simulink model "MUDV_projekt"  (R2023a)
settings: Solver=ode23tb  StartTime=0.0  StopTime=20  FixedStep=.001  RelTol=2e-1  EnableMultiTasking=on
InitFcn:
  | v=version('-release');
  | if (str2num(v(1:end-1)) > 2021)
  | set_param('MUDV_projekt/Passenger Vehicle/Body, suspension and tires/MacPherson Front Suspension Solid Axle Rear Suspension/independent Suspensions - MacPherson','NumWhlsByAxl','2');
  | set_param('MUDV_projekt/Passenger Vehicle/Body, suspension and tires/MacPherson Front Suspension Solid Axle Rear Suspension/Solid Axle Suspension - Coil Spring','NumWhlsByAxl','2');
  | end
StartFcn:
  | %tic
StopFcn:
  | %toc
model workspace (MAT data in the model file):
  AxlIxx = 62.3745166667
  AxlM = 160
  Cps = 2
  Cz = 5565.2246438
  CzWhlAxl = 11490.971257
  DCT_Param : object (value not decoded)
  DLCXref = [0 7.35 7.45 18 33 33.5 45 50 60]
  DLCYref = [0 0 -4.5 -4.35 -3.75 1.25 1 0 0]
  EngRevLim = 7000
  F0z = [2886 2907]
  F0zWhlAxl = 2907
  Hmax = 0.25
  Kz = 52451.0065793
  KzWhlAxl = 138031.612078
  NCyl = 6
  Pedal_Positions = [0.1 0.4 0.5 0.9]
  Pstd = 101325
  Rair = 287
  SUS : object (value not decoded)
  Sig : Simulink.Signal (value not decoded)
  Sig1 : Simulink.Signal (value not decoded)
  Trans : object (value not decoded)
  Tstd = 293.15
  VEH : object (value not decoded)
  Vd = 0.00346
  WH : Mass (value not decoded)
  dt3D = 0.05
  f_air = [0 0 0 0 0 0 0 0 0 0 0 0 ... (256 elements, 16x16)]
  f_co = [0 0 0 0 0 0 0 0 0 0 0 0 ... (256 elements, 16x16)]
  f_co2 = [0 0 0 0 0 0 0 0 0 0 0 0 ... (256 elements, 16x16)]
  f_eff = [352.135682859 352.135682859 320.724378192 303.655312657 295.930136708 291.240087194 291.240271258 291.240312459 291.240275452 291.240198499 291.240100781 291.240018769 ... (256 elements, 16x16)]
  f_fuel = [0 0 0 0 0 0 0 0 0 0 0 0 ... (256 elements, 16x16)]
  f_hc = [0 0 0 0 0 0 0 0 0 0 0 0 ... (256 elements, 16x16)]
  f_nox = [0 0 0 0 0 0 0 0 0 0 0 0 ... (256 elements, 16x16)]
  f_pm = [0 0 0 0 0 0 0 0 0 0 0 0 ... (256 elements, 16x16)]
  f_susp_axl_bp = [1 2]
  f_susp_dz_bp = [-0.325022776267 -0.315022776267 -0.305022776267 -0.205022776267 -0.105022776267 -0.00502277626717 0.0949772237328 0.194977223733 0.204977223733 0.214977223733]
  f_susp_dzdot_bp = [-3 -0.3 -0.2 -0.1 0 0.1 0.2 0.3 3]
  f_susp_fmz = [-144070.391448 -93629.24037 -75929.1118915 -20630.5828179 -15385.48216 -10140.3815021 -4895.28084414 349.819813785 -31916.3973792 18437.6709544 -83996.1993354 -33555.0482577 ... (43920 elements, 10x9x61x2x4)]
  f_susp_geom = [0 0 0 0 0 0 0 0 0 0 0 0 ... (3660 elements, 10x61x2x3)]
  f_susp_strgdelta_bp = [-0.523598775598 -0.506145483078 -0.488692190558 -0.471238898038 -0.453785605519 -0.436332312999 -0.418879020479 -0.401425727959 -0.383972435439 -0.366519142919 -0.349065850399 -0.331612557879 ... (61 elements, 1x61)]
  f_tbrake = [0 76.8593923996 105.140482948 131.533638111 157.926793274 176.658631717 176.65727296 176.656856686 176.656879077 176.657093756 176.657404516 176.65772406 ... (256 elements, 16x16)]
  f_tbrake_n_bpt = [0 649.519052838 912.419621844 1175.32019085 1438.22075986 1701.12132886 1964.02189787 2226.92246687 2489.82303588 2752.72360489 3015.62417389 3278.5247429 ... (16 elements, 1x16)]
  f_tbrake_t_bpt = [0 34.6410161514 61.0341713143 87.4273264773 113.82048164 140.213636803 166.606791966 192.999947129 219.393102292 245.786257455 272.179412618 298.572567781 ... (16 elements, 1x16)]
  f_texh = [766.752464599 766.752464599 786.17542386 801.679939032 884.591982581 910.574397722 910.571871054 910.570774534 910.570601632 910.570821151 910.571247242 910.571639815 ... (256 elements, 16x16)]
  f_twc_eff_co = [0.17 0.25 0.45 0.99 0.99 0.99 0.99]
  f_twc_eff_hc = [0.21 0.375 0.75 0.98 0.98 0.98 0.98]
  f_twc_eff_lam = [0.909090909 0.944055944 0.979020979 1 1.013986014 1.048951049 1.083916084]
  f_twc_eff_nox = [0.98 0.98 0.98 0.97 0.05 0.02 0]
  numWheel = 4
symbols that are objects in the model workspace (value not decoded): VEH
libraries: sharedtransform x3, autolibutils x3, sim3dlib x2, vehdynlibsuspension x2, shared6dof x2, vehdynlibeom x1, vehdynlibtirecommon x1, vehdynlibtire x1, vehdynlibsteering x1, vehdynlibsens x1, sim3dautolib x1
(part 2 of 4)

== system MUDV_projekt/ Reference Generator  ==
  VehFdbk : Inport
  Add : Sum
  Bus Creator1 : BusCreator  Inputs=3
  Bus Selector : BusSelector  OutputSignals=Body.InertFrm.Cg.Disp.X
  DLC Reference : MATLAB Function  TreatAsAtomicUnit=on
  Manual Switch : ManualSwitch  CurrentSetting=0
  Rate Limiter : RateLimiter  RisingSlewLimit=10  FallingSlewLimit=-10  SampleTimeMode=inherited
  Scope : Scope
  Unit Delay : UnitDelay  SampleTime=1e-3  HasFrameUpgradeWarning=on
  X_offset : Constant  Value=30
  Y_offset : Constant  Value=0.2
  "km/h -> m/s" : Gain  Gain=1/3.6
  vxRef : Step  Time=0.1  After=50  SampleTime=0
  vxRef1 : Step  Time=0.1  After=20  SampleTime=10
  VehRef : Outport
  wires:
  Bus Creator1/1 -> VehRef/1
  DLC Reference/2(YRef) -> Bus Creator1/3  "LtrlRef"
  DLC Reference/1(YawRef) -> Bus Creator1/2  "YawRef"
  VehFdbk/1 -> Bus Selector/1
  Bus Selector/1 -> Unit Delay/1  "<X>"
  Y_offset/1 -> DLC Reference/3(Y_offset)
  "km/h -> m/s"/1 -> Scope/1, Bus Creator1/1  "LngRef"
  Unit Delay/1 -> DLC Reference/1(X)
  Rate Limiter/1 -> "km/h -> m/s"/1
  X_offset/1 -> DLC Reference/2(X_offset)
  Manual Switch/1 -> Rate Limiter/1
  vxRef/1 -> Manual Switch/2, Add/2
  Add/1 -> Manual Switch/1
  vxRef1/1 -> Add/1

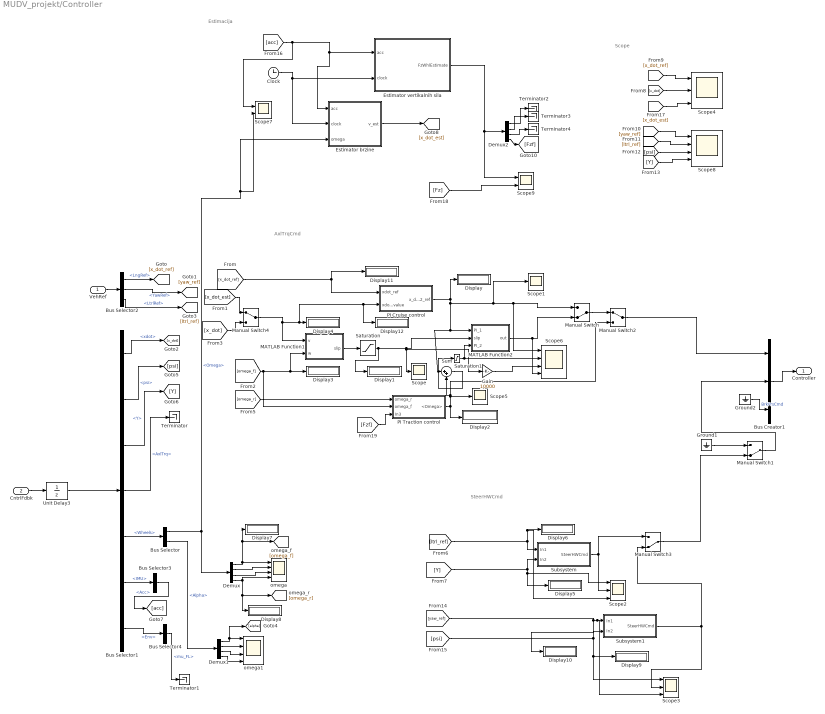
== system MUDV_projekt/Controller ==
  note: Estimacija
  note: Scope
  note: AxlTrqCmd
  note: SteerHWCmd
  VehRef : Inport
  CntrlFdbk : Inport  Port=2
  Bus Creator1 : BusCreator  Inputs=3
  Bus Selector : BusSelector  OutputSignals=Omega,Alpha
  Bus Selector1 : BusSelector  OutputSignals=xdot,psi,Y,AxlTrq,Wheels,IMU,Env
  Bus Selector2 : BusSelector  OutputSignals=LngRef,YawRef,LtrlRef
  Bus Selector3 : BusSelector  OutputSignals=Acc
  Bus Selector4 : BusSelector  OutputSignals=Gnd.mu.mu_FL
  Clock : Clock
  Demux : Demux
  Demux1 : Demux
  Demux2 : Demux
  Display{,1..12} (13 alike) : Display
  Estimator brzine : MATLAB Function  TreatAsAtomicUnit=on
  Estimator vertikalnih sila : MATLAB Function  TreatAsAtomicUnit=on
  Gain : Gain  Gain=10000
  Ground1 : Ground
  Ground2 : Ground
  MATLAB Function1 : MATLAB Function  TreatAsAtomicUnit=on
  MATLAB Function2 : MATLAB Function  TreatAsAtomicUnit=on
  Manual Switch : ManualSwitch  CurrentSetting=0
  Manual Switch1 : ManualSwitch  CurrentSetting=0
  Manual Switch2 : ManualSwitch
  Manual Switch3 : ManualSwitch  CurrentSetting=0
  Manual Switch4 : ManualSwitch
  PI Cruise control : Subsystem
  PI Traction control : Subsystem
  Saturation : Saturate  UpperLimit=1  LowerLimit=0
  Saturation1 : Saturate  UpperLimit=1500  LowerLimit=-1500
  Scope : Scope
  Scope1 : Scope
  Scope2 : Scope  NumInputPorts=3
  Scope3 : Scope  NumInputPorts=3
  Scope4 : Scope  NumInputPorts=3
  Scope5 : Scope
  Scope6 : Scope  NumInputPorts=4
  Scope7 : Scope  NumInputPorts=2
  Scope8 : Scope  NumInputPorts=4
  Scope9 : Scope  NumInputPorts=2
  Subsystem : Subsystem
  Subsystem1 : Subsystem
  Sum : Sum  Inputs=|++
  Terminator{,1..4} (5 alike) : Terminator
  Unit Delay3 : UnitDelay  SampleTime=1e-3  HasFrameUpgradeWarning=on
  omega : Scope  NumInputPorts=4
  omega1 : Scope  NumInputPorts=4
  Controller : Outport
  wires:
  Bus Creator1/1 -> Controller/1
  Bus Selector1/4 -> Terminator/1  "<AxlTrq>"
  Bus Selector1/6 -> Bus Selector3/1  "<IMU>"
  Bus Selector1/7 -> Bus Selector4/1  "<Env>"
  Bus Selector1/5 -> Bus Selector/1  "<Wheels>"
  VehRef/1 -> Bus Selector2/1
  Bus Selector1/2 -> [psi]  "<psi>"
  CntrlFdbk/1 -> Unit Delay3/1
  Unit Delay3/1 -> Bus Selector1/1
  Bus Selector2/3 -> [ltrl_ref]  "<LtrlRef>"
  Bus Selector1/1 -> [x_dot]  "<xdot>"
  Bus Selector3/1 -> [acc]  "<Acc>"
  PI Cruise control/1(x_dot_2_ref) -> Sum/1, MATLAB Function2/1(PI_1), Scope1/1, Scope6/1, Manual Switch/1, Display/1
  Bus Selector2/1 -> [x_dot_ref]  "<LngRef>"
  MATLAB Function2/1(out) -> Scope6/4, Manual Switch/2
  Demux/1 -> Display7/1, [omega_f], omega/1
  Demux/2 -> omega/2
  Demux/3 -> omega/3
  Bus Selector/1 -> Scope7/2, Estimator brzine/3(omega), Demux/1  "<Omega>"
  [omega_f] -> PI Traction control/2(omega_f), MATLAB Function1/2(w), Display3/1
  [omega_r] -> PI Traction control/1(omega_r)
  PI Traction control/1(<Omega>) -> Manual Switch2/2, Sum/2, Scope5/1, Display2/1
  MATLAB Function1/1(slip) -> Saturation/1
  Bus Selector2/2 -> [yaw_ref]  "<YawRef>"
  [ltrl_ref] -> Subsystem/1(In1), Scope2/3, Display6/1
  [Y] -> Subsystem/2(In2), Display5/1, Scope2/1
  Ground2/1 -> Bus Creator1/3  "BrkPrsCmd"
  Bus Selector/2 -> Demux1/1  "<Alpha>"
  Demux1/1 -> [alpha], omega1/1
  Demux1/2 -> omega1/2
  Demux1/3 -> omega1/3
  Demux1/4 -> omega1/4
  Ground1/1 -> Manual Switch1/1
  Subsystem/1(SteerHWCmd) -> Manual Switch3/1, Scope2/2
  Manual Switch1/1 -> Bus Creator1/2
  Demux/4 -> Display8/1, [omega_r], omega/4
  [x_dot_ref] -> Scope4/1
  [x_dot] -> Scope4/2
  Manual Switch/1 -> Manual Switch2/1
  Manual Switch2/1 -> Bus Creator1/1
  Bus Selector1/3 -> [Y]  "<Y>"
  [Y] -> Scope8/4
  [psi] -> Scope8/3
  [ltrl_ref] -> Scope8/2
  [yaw_ref] -> Scope8/1
  [psi] -> Subsystem1/2(In2), Scope3/1, Display9/1
  [yaw_ref] -> Scope3/3, Subsystem1/1(In1), Display10/1
  Subsystem1/1(SteerHWCmd) -> Scope3/2, Manual Switch3/2
  Manual Switch3/1 -> Manual Switch1/2
  Estimator vertikalnih sila/1(FzWhlEstimate) -> Demux2/1, Scope9/1
  Clock/1 -> Estimator brzine/2(clock), Estimator vertikalnih sila/2(clock)
  [acc] -> Scope7/1, Estimator brzine/1(acc), Estimator vertikalnih sila/1(acc)
  Estimator brzine/1(v_est) -> [x_dot_est]
  [x_dot_est] -> Scope4/3
  Saturation/1 -> MATLAB Function2/2(slip), Scope/1, Gain/1, Display1/1
  [Fz] -> Scope9/2
  Demux2/1 -> Terminator2/1
  Demux2/4 -> [Fzf]
  Demux2/3 -> Terminator4/1
  Demux2/2 -> Terminator3/1
  [Fzf] -> PI Traction control/3(In3)
  Bus Selector4/1 -> Terminator1/1  "<mu_FL>"
  Gain/1 -> Scope6/3
  Sum/1 -> Saturation1/1
  Saturation1/1 -> Scope6/2, MATLAB Function2/3(PI_2)
  [x_dot_ref] -> Display11/1, PI Cruise control/1(xdot_ref)
  [x_dot_est] -> Manual Switch4/1
  [x_dot] -> Manual Switch4/2
  Manual Switch4/1 -> MATLAB Function1/1(v), Display12/1, PI Cruise control/2(xdot_value), Display4/1

== system MUDV_projekt/Environment ==
  Bus Creator1 : BusCreator  Inputs=2
  Constant3 : Constant  Value=0
  Constant4 : Constant  Value=0
  Constant5 : Constant  Value=0
  Demux : Demux
  Friction : Constant  Value=[1; 1; 1; 1]*0.6
  Ground Feedback : Subsystem  Variant=on  VariantControlMode=label  LabelModeActiveChoice=0
  Scope : Scope  NumInputPorts=4
  Vector Concatenate : Concatenate  NumInputs=3
  Out1 : Outport
  wires:
  Bus Creator1/1 -> Out1/1
  Constant5/1 -> Vector Concatenate/3  "Z"
  Constant4/1 -> Vector Concatenate/2  "Y"
  Vector Concatenate/1 -> Bus Creator1/1  "Wind"
  Friction/1 -> Demux/1, Ground Feedback/1(Friction)
  Constant3/1 -> Vector Concatenate/1  "X"
  Ground Feedback/1(Ground) -> Bus Creator1/2  "Gnd"
  Demux/2 -> Scope/2
  Demux/4 -> [friction], Scope/3
  Demux/3 -> Scope/4
  Demux/1 -> Scope/1

== system MUDV_projekt/Passenger Vehicle ==
  Controller : Inport
  Env : Inport  Port=2
  "Body, suspension and tires" : Subsystem
  Chassis Input : Subsystem
  Chassis Output : Subsystem
  Driveline : Subsystem
  Driveline Input : Subsystem
  Driveline Output : Subsystem
  Out Bus Element4 : Outport  PortName=VehFdbk  Element=Body
  Out Bus Element5 : Outport  PortName=VehFdbk  Element=Wheels
  Out Bus Element1 : Outport  PortName=VehFdbk  Element=Driveline
  wires:
  Env/1 -> Chassis Input/1(Env)
  Chassis Input/1(Wind) -> "Body, suspension and tires"/1(WindXYZ)
  Chassis Input/2(Gnd) -> "Body, suspension and tires"/2(Ground)
  Chassis Input/3(mu) -> "Body, suspension and tires"/3(Friction)
  Chassis Input/4(WhlAng) -> "Body, suspension and tires"/4(WhlAng)
  Chassis Input/5(AxlTrq) -> "Body, suspension and tires"/5(AxlTrq)
  Chassis Input/6(BrkPrs) -> "Body, suspension and tires"/6(BrkPrs)
  [Driveline] -> Chassis Input/2(Driveline)
  "Body, suspension and tires"/2(Wheels) -> Chassis Output/2(Wheels)
  "Body, suspension and tires"/1(Veh) -> Chassis Output/1(Veh)
  Chassis Output/2(WheelsFdbk) -> Out Bus Element5/1
  Chassis Output/1(VehFdbk) -> Out Bus Element4/1
  Driveline Input/2(AxlTrqCmd) -> Driveline/2(AxlTrqCmd)
  Driveline Input/1(Steer) -> Driveline/1(SteerHWCmd)
  Driveline Input/3(BrkPrsCmd) -> Driveline/3(BrkPrsCmd)
  Driveline Output/1(Driveline) -> Out Bus Element1/1, [Driveline]  "Driveline"
  Driveline/2(AxlTrq) -> Driveline Output/2(AxlTrq)
  Driveline/1(WhlAng) -> Driveline Output/1(WhlAng)
  Driveline/3(BrkPrs) -> Driveline Output/3(BrkPrs)
  Controller/1 -> Driveline Input/1(Controller)

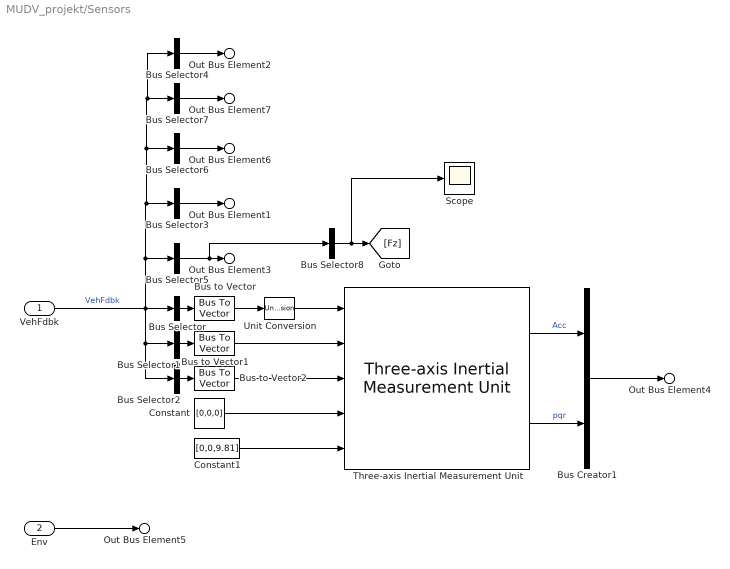
== system MUDV_projekt/Sensors ==
  VehFdbk : Inport
  Env : Inport  Port=2
  Bus Creator1 : BusCreator  Inputs=2
  Bus Selector : BusSelector  OutputSignals=Body.BdyFrm.Cg.Acc.ax,Body.BdyFrm.Cg.Acc.ay,Body.BdyFrm.Cg.Acc.az  OutputAsBus=on
  Bus Selector1 : BusSelector  OutputSignals=Body.BdyFrm.Cg.AngVel.p,Body.BdyFrm.Cg.AngVel.q,Body.BdyFrm.Cg.AngVel.r  OutputAsBus=on
  Bus Selector2 : BusSelector  OutputSignals=Body.BdyFrm.Cg.AngAcc.pdot,Body.BdyFrm.Cg.AngAcc.qdot,Body.BdyFrm.Cg.AngAcc.rdot  OutputAsBus=on
  Bus Selector3 : BusSelector  OutputSignals=Driveline.AxlTrq  OutputAsBus=on
  Bus Selector4 : BusSelector  OutputSignals=Body.BdyFrm.Geom.Vel.xdot  OutputAsBus=on
  Bus Selector5 : BusSelector  OutputSignals=Wheels.TireFrame.Fz,Driveline.BrkPrs,Wheels.TireFrame.Kappa,Wheels.TireFrame.Alpha,Wheels.TireFrame.Omega  OutputAsBus=on
  Bus Selector6 : BusSelector  OutputSignals=Body.InertFrm.Geom.Disp.Y  OutputAsBus=on
  Bus Selector7 : BusSelector  OutputSignals=Body.InertFrm.Cg.Ang.psi  OutputAsBus=on
  Bus Selector8 : BusSelector  OutputSignals=Fz  OutputAsBus=on
  Bus to Vector : BusToVector
  Bus to Vector1 : BusToVector
  Bus to Vector2 : BusToVector
  Constant : Constant  Value=[0,0,0]
  Constant1 : Constant  Value=[0,0,9.81]
  Scope : Scope
  Three-axis Inertial Measurement Unit : vehdynlibsens/Three-axis Inertial Measurement Unit  units=Metric (MKS)  imu=[0 0 0]  i_Ts=0  dtype_a=off  w_a=190  z_a=0.707  a_sf_cc=[1 0 0; 0 1 0; 0 0 1]  a_bias=[0 0 0]  a_sat="[-inf  -inf  -inf  inf inf inf]"  dtype_g=off  w_g=190  z_g=0.707  g_sf_cc=[1 0 0; 0 1 0; 0 0 1]  g_bias=[0 0 0]  g_sens=[0 0 0]  g_sat="[-inf  -inf  -inf  inf inf inf]"  i_rand=on  i_seeds=[23093 23094 23095 23096 23097 23098]  i_pow=[0.001 0.001 0.001 0.0001 0.0001 0.0001]  aMode=2
  Unit Conversion : UnitConversion
  Out Bus Element3 : Outport  PortName=CntrlRx  Element=Wheels
  Out Bus Element4 : Outport  PortName=CntrlRx  Element=IMU
  Out Bus Element5 : Outport  PortName=CntrlRx  Element=Env
  Out Bus Element1 : Outport  PortName=CntrlRx  Element=AxlTrq
  Out Bus Element2 : Outport  PortName=CntrlRx  Element=xdot
  Out Bus Element6 : Outport  PortName=CntrlRx  Element=Y
  Out Bus Element7 : Outport  PortName=CntrlRx  Element=psi
  wires:
  VehFdbk/1 -> Bus Selector/1, Bus Selector2/1, Bus Selector1/1, Bus Selector4/1, Bus Selector7/1, Bus Selector6/1, Bus Selector3/1, Bus Selector5/1  "VehFdbk"
  Bus Creator1/1 -> Out Bus Element4/1
  Three-axis Inertial Measurement Unit/1 -> Bus Creator1/1  "Acc"
  Three-axis Inertial Measurement Unit/2 -> Bus Creator1/2  "pqr"
  Bus Selector/1 -> Bus to Vector/1
  Bus to Vector/1 -> Unit Conversion/1
  Bus Selector1/1 -> Bus to Vector1/1
  Bus to Vector1/1 -> Three-axis Inertial Measurement Unit/2
  Env/1 -> Out Bus Element5/1
  Bus Selector2/1 -> Bus to Vector2/1
  Bus to Vector2/1 -> Three-axis Inertial Measurement Unit/3
  Constant/1 -> Three-axis Inertial Measurement Unit/4
  Constant1/1 -> Three-axis Inertial Measurement Unit/5
  Unit Conversion/1 -> Three-axis Inertial Measurement Unit/1
  Bus Selector5/1 -> Bus Selector8/1, Out Bus Element3/1
  Bus Selector3/1 -> Out Bus Element1/1
  Bus Selector6/1 -> Out Bus Element6/1
  Bus Selector7/1 -> Out Bus Element7/1
  Bus Selector4/1 -> Out Bus Element2/1
  Bus Selector8/1 -> Scope/1, [Fz]

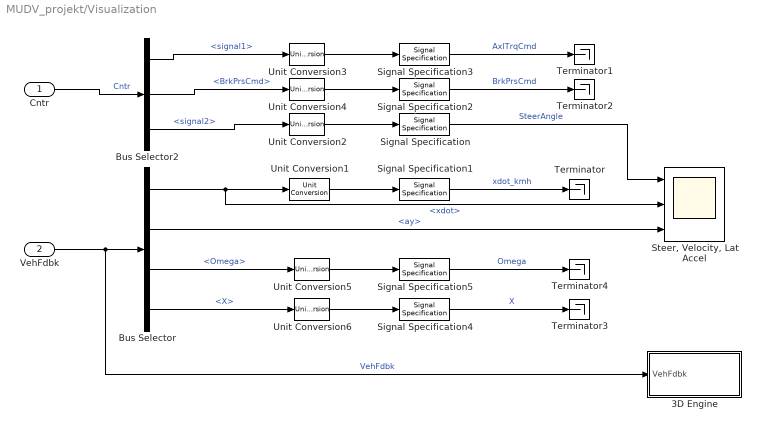
== system MUDV_projekt/Visualization ==
  Cntr : Inport
  VehFdbk : Inport  Port=2
  3D Engine : Subsystem  Variant=on  mask(3D Engine){engine3D=Disabled, use3DOp=off, SceneDesc=Straight road, dt3D=.03, defaultPos=User-specified, X_o=0, Y_o=0.2, Z_o=0, phi_o=0, theta_o=0, psi_o=0}
      mask prompts: engine3D "3D Engine"; use3DOp "Use default operating point"; SceneDesc "Scene:"; dt3D "Engine frame rate, dt3D [s]:"; X_o "Initial longitudinal position, X_o [m]:"; Y_o "Initial lateral position, Y_o [m]:"; Z_o "Initial vertical position, Z_o [m]:"; phi_o "Initial roll angle, phi_o [rad]:"; theta_o "Initial pitch angle, theta_o [rad]:"; psi_o "Initial yaw angle, psi_o [rad]:"
      mask help: This subsystem contains the interface blocks which permit the display of the vehicle in the 3D virtual environment. Enable it to view the simulation progress, disable it to inhibit the display.
      mask init:
      | switch get_param(gcb,'engine3D')
      |     case 'Disabled'
      |         try
      |             set_param([bdroot '/Environment/Ground Feedback'],'OverrideUsingVariant','0');
      |         catch
      |             disp('Warning: No ground feedback sensor not set')
      |         end
      |         try
      |             if strcmp(get_param(gcb,'use3DOp'),'on') && strcmp(get_param('DLCReferenceApplication/Lane Change Reference Generator','ssMode'),'Resume from a workspace variable')
      |                 set_param('DLCReferenceApplication/Lane Change Reference Generator','ssVar','dlcSS35mph');
      |             end
      |         catch
      |              disp('Warning: Lane Change Reference Generator not found. Steady state operating point not set')
      |         end
      |     case 'Enabled'
      |         try
      |             set_param([bdroot '/Environment/Ground Feedback'],'OverrideUsingVariant','1');            
      |         catch
      |             disp('Warning: No ground feedback sensor not set')
      |         end
      |         try
      |             if strcmp(get_param(gcb,'use3DOp'),'on') && strcmp(get_param('DLCReferenceApplication/Lane Change Reference Generator','ssMode'),'Resume from a workspace variable')
      |                 set_param('DLCReferenceApplication/Lane Change Reference Generator','ssVar','dlcSS35mph3D');
      |             end
      |         catch
      |              disp('Warning: Lane Change Reference Generator not found. Steady state operating point not set')
      |         end
      |     otherwise
      | end
      settings: AttributesFormatString=|
      | %<SceneDesc>
      | %<engine3D>
      mask Help: eval('vdynblkshelp(''vdynblks3dengine'')');
      mask TypeOptions engine3D: Enabled | Disabled
      mask TypeOptions SceneDesc: 3D Engine/Simulation 3D Scene Configuration/SceneDesc
      mask Callback SceneDesc:
      | defaultStatus = get_param(gcb,'defaultPos');
      | if strcmp(defaultStatus,'Recommended for scene')
      | sceneType = get_param(gcb,'SceneDesc');
      | switch sceneType
      |     case 'Straight road'
      |         set_param(gcb,'X_o', '-118')
      |         set_param(gcb,'Y_o', '3.125')
      |         set_param(gcb,'Z_o', '0')
      |         set_param(gcb,'phi_o', '0')
      |         set_param(gcb,'theta_o', '0')
      |         set_param(gcb,'psi_o', '0')
      |     case 'Curved road'
      |         set_param(gcb,'X_o', '0.2')
      |         set_param(gcb,'Y_o', '-1605.0')
      |         set_param(gcb,'Z_o', '0')
      |         set_param(gcb,'phi_o', '0')
      |         set_param(gcb,'theta_o', '0')
      |         set_param(gcb,'psi_o', '-156*pi/180')
      |     case 'Parking lot'
      |         set_param(gcb,'X_o', '-104.0')
      |         set_param(gcb,'Y_o', '-9.7')
      |         set_param(gcb,'Z_o', '0')
      |         set_param(gcb,'phi_o', '0')
      |         set_param(gcb,'theta_o', '0')
      |         set_param(gcb,'psi_o', '0')
      |     case 'Double lane change'
      |         set_param(gcb,'X_o', '0')
      |         set_param(gcb,'Y_o', '3.125')
      |         set_param(gcb,'Z_o', '0')
      |         set_param(gcb,'phi_o', '0')
      |         set_param(gcb,'theta_o', '0')
      |         set_param(gcb,'psi_o', '0')
      |     case 'Open surface'
      |         set_param(gcb,'X_o', '0')
      |         set_param(gcb,'Y_o', '0')
      |         set_param(gcb,'Z_o', '0')
      |         set_param(gcb,'phi_o', '0')
      |         set_param(gcb,'theta_o', '0')
      |         set_param(gcb,'psi_o', '0')
      |     case 'US highway'
      |         set_param(gcb,'X_o', '3592.00')
      |         set_param(gcb,'Y_o', '2617.00')
      |         set_param(gcb,'Z_o', '-1.0')
      |         set_param(gcb,'phi_o', '0')
      |         set_param(gcb,'theta_o', '0')
      |         set_param(gcb,'psi_o', '0')
      |     case 'US city block'
      |         set_param(gcb,'X_o', '-125.19')
      |         set_param(gcb,'Y_o', '1.65')
      |         set_param(gcb,'Z_o', '-0.04')
      |         set_param(gcb,'phi_o', '0')
      |         set_param(gcb,'theta_o', '0')
      |         set_param(gcb,'psi_o', '0')
      |     case 'Large parking lot'
      |         set_param(gcb,'X_o', '45.0')
      |         set_param(gcb,'Y_o', '54.7')
      |         set_param(gcb,'Z_o', '0.0')
      |         set_param(gcb,'phi_o', '0')
      |         set_param(gcb,'theta_o', '0')
      |         set_param(gcb,'psi_o', '-pi/2')
      |     case 'Virtual Mcity'
      |         set_param(gcb,'X_o', '-26.0')
      |         set_param(gcb,'Y_o', '76.0')
      |         set_param(gcb,'Z_o', '0.0')
      |         set_param(gcb,'phi_o', '0')
      |         set_param(gcb,'theta_o', '0')
      |         set_param(gcb,'psi_o', '-40*pi/180')
      |     otherwise
      |         set_param(gcb,'X_o', '0')
      |         set_param(gcb,'Y_o', '0')
      |         set_param(gcb,'Z_o', '0')
      |         set_param(gcb,'phi_o', '0')
      |         set_param(gcb,'theta_o', '0')
      |         set_param(gcb,'psi_o', '0')
      | end
      | end
      mask TypeOptions defaultPos: Recommended for scene | User-specified
      mask DialogControl engineConfig Prompt: 3D Engine Settings
      mask DialogControl posSetup Prompt: Initial vehicle position
      mask DialogControl posSetupDesc Prompt: To use these initial vehicle positions, first Apply the initial values and then click Update the model workspaces with the initial values.
      mask DialogControl setModelPos Prompt: Update model workspaces with initial values
      mask DialogControl setModelPos Callback:
      | if strcmp(get_param(bdroot(gcb),'SimulationStatus'),'stopped')
      |     sceneType = get_param(gcb,'SceneDesc');
      |     rootModel = bdroot(gcb);
      |     ws = get_param(rootModel, 'modelworkspace');
      |     VEH = getVariable(ws,'VEH');
      |     ParamList={'X_o',[1,1],{};'Y_o',[1,1],{};'Z_o',[1,1],{};'phi_o',[1,1],{'gte',-pi/2;'lte',pi/2};'theta_o',[1,1],{'gte',-pi/2;'lte',pi/2};'psi_o',[1,1],{'gte',-2*pi;'lte',2*pi}};
      |     paramStruct = autoblkscheckparams(gcb, '3D Engine',ParamList);
      |     VEH.InitialLongPosition = paramStruct.X_o;
      |     VEH.InitialLatPosition = paramStruct.Y_o;
      |     VEH.InitialVertPosition = paramStruct.Z_o;
      |     VEH.InitialRollAngle = paramStruct.phi_o;
      |     VEH.InitialPitchAngle = paramStruct.theta_o;
      |     VEH.InitialYawAngle = paramStruct.psi_o;
      |     assignin(ws,'VEH',VEH);
      |     modelList = {'PassVeh14DOF','PassVeh7DOF'};
      |     for idx =1:length(modelList)
      | %         try
      |             load_system(modelList{idx});
      |             ws = get_param(modelList{idx}, 'modelworkspace');
      |             assignin(ws,'VEH',VEH);
      |             save_system(modelList{idx});
      |             close_system(modelList{idx});
      | %         catch
      | %             disp(['Cannot find ' modelList{idx}])
      | %         end
      |     end
      | end
      mask Display: disp('3D Engine')
  Bus Selector : BusSelector  OutputSignals=Body.BdyFrm.Cg.Vel.xdot,Body.BdyFrm.Cg.Acc.ay,Wheels.TireFrame.Omega,Body.InertFrm.Cg.Disp.X
  Bus Selector2 : BusSelector  OutputSignals=signal1,BrkPrsCmd,signal2
  Signal Specification : SignalSpecification  Unit=deg
  Signal Specification1 : SignalSpecification  Unit=km/h
  Signal Specification2 : SignalSpecification  Unit=Pa
  Signal Specification3 : SignalSpecification  Unit=N*m
  Signal Specification4 : SignalSpecification  Unit=m
  Signal Specification5 : SignalSpecification  Unit=deg/s
  "Steer, Velocity, Lat Accel" : Scope  NumInputPorts=3
  Terminator{,1..4} (5 alike) : Terminator
  Unit Conversion{1..6} (6 alike) : UnitConversion
  wires:
  Signal Specification/1 -> "Steer, Velocity, Lat Accel"/1  "SteerAngle"
  Bus Selector/2 -> "Steer, Velocity, Lat Accel"/3  "<ay>"
  Bus Selector/1 -> "Steer, Velocity, Lat Accel"/2, Unit Conversion1/1  "<xdot>"
  Unit Conversion2/1 -> Signal Specification/1
  Unit Conversion1/1 -> Signal Specification1/1
  Signal Specification1/1 -> Terminator/1  "xdot_kmh"
  VehFdbk/1 -> 3D Engine/1(VehFdbk), Bus Selector/1  "VehFdbk"
  Bus Selector2/3 -> Unit Conversion2/1  "<signal2>"
  Cntr/1 -> Bus Selector2/1  "Cntr"
  Bus Selector2/1 -> Unit Conversion3/1  "<signal1>"
  Bus Selector2/2 -> Unit Conversion4/1  "<BrkPrsCmd>"
  Unit Conversion4/1 -> Signal Specification2/1
  Unit Conversion3/1 -> Signal Specification3/1
  Signal Specification3/1 -> Terminator1/1  "AxlTrqCmd"
  Signal Specification2/1 -> Terminator2/1  "BrkPrsCmd"
  Bus Selector/3 -> Unit Conversion5/1  "<Omega>"
  Unit Conversion5/1 -> Signal Specification5/1
  Signal Specification5/1 -> Terminator4/1  "Omega"
  Bus Selector/4 -> Unit Conversion6/1  "<X>"
  Unit Conversion6/1 -> Signal Specification4/1
  Signal Specification4/1 -> Terminator3/1  "X"

== system MUDV_projekt/Controller/PI Cruise control ==
  xdot_ref : Inport
  xdot_value : Inport  Port=2
  Add : Sum
  Integrator : Integrator
  Ki : Gain  Gain=8
  Kp : Gain  Gain=1000
  Saturation : Saturate  UpperLimit=1500  LowerLimit=-1500
  Sum1 : Sum  Inputs=|+-
  x_dot_2_ref : Outport
  wires:
  Kp/1 -> Add/1
  Integrator/1 -> Ki/1
  Sum1/1 -> Integrator/1, Kp/1  "x_dot-error"
  Ki/1 -> Add/2
  xdot_value/1 -> Sum1/2
  xdot_ref/1 -> Sum1/1
  Saturation/1 -> x_dot_2_ref/1
  Add/1 -> Saturation/1

== system MUDV_projekt/Controller/PI Traction control ==
  omega_r : Inport
  omega_f : Inport  Port=2
  In3 : Inport  Port=3
  Add : Sum
  Add1 : Sum  Inputs=-+
  Gain : Gain  Gain=1/(1-0.1)
  Gain1 : Gain  Gain=0.007*0.3*0.7
  Integrator : Integrator
  Ki : Gain  Gain=0
  Kp : Gain  Gain=100
  Kp1 : Gain  Gain=0
  Scope : Scope
  Scope1 : Scope  NumInputPorts=4
  Scope2 : Scope
  Sum : Sum  Inputs=|+-
  Sum1 : Sum  Inputs=|++
  Sum2 : Sum  Inputs=|++
  <Omega> : Outport
  wires:
  omega_r/1 -> Scope1/4, Gain/1
  Gain/1 -> Scope1/1, Sum/1
  Kp/1 -> Add/1
  Sum1/1 -> Add1/2, Scope2/1, <Omega>/1, Add1/1
  omega_f/1 -> Scope1/2, Sum/2
  Add/1 -> Sum1/1
  In3/1 -> Gain1/1
  Gain1/1 -> Scope/1, Sum1/2
  Sum/1 -> Scope1/3, Ki/1, Kp/1  "error"
  Integrator/1 -> Add/2
  Ki/1 -> Sum2/1
  Sum2/1 -> Integrator/1
  Add1/1 -> Kp1/1
  Kp1/1 -> Sum2/2

== system MUDV_projekt/Controller/Subsystem ==
  In1 : Inport
  In2 : Inport  Port=2
  Add : Sum  Inputs=+++
  Add1 : Sum  Inputs=-+
  Derivative : Derivative
  Gain1 : Gain  Gain=18
  Integrator : Integrator
  Ki : Gain
  Ki1 : Gain
  Kp : Gain  Gain=10
  Kp1 : Gain  Gain=10
  Manual Switch : ManualSwitch  CurrentSetting=0
  Saturation : Saturate  UpperLimit=5  LowerLimit=-5
  Sum : Sum  Inputs=|+-
  Sum1 : Sum  Inputs=|++
  SteerHWCmd : Outport
  wires:
  In1/1 -> Manual Switch/1, Sum/1
  Sum/1 -> Kp1/1, Ki/1, Kp/1  "error"
  Kp/1 -> Add/1
  In2/1 -> Sum/2
  Gain1/1 -> Manual Switch/2
  Manual Switch/1 -> SteerHWCmd/1
  Add/1 -> Add1/1, Saturation/1
  Saturation/1 -> Add1/2, Gain1/1
  Ki/1 -> Sum1/1
  Sum1/1 -> Integrator/1
  Integrator/1 -> Add/3
  Ki1/1 -> Sum1/2
  Add1/1 -> Ki1/1
  Kp1/1 -> Derivative/1
  Derivative/1 -> Add/2

== system MUDV_projekt/Controller/Subsystem1 ==
  In1 : Inport
  In2 : Inport  Port=2
  Add : Sum  Inputs=+++
  Add1 : Sum  Inputs=-+
  Derivative : Derivative
  Gain1 : Gain  Gain=18
  Integrator : Integrator
  Ki : Gain  Gain=0
  Ki1 : Gain  Gain=0
  Kp : Gain  Gain=1.6
  Kp1 : Gain
  Manual Switch : ManualSwitch  CurrentSetting=0
  Saturation : Saturate  UpperLimit=pi  LowerLimit=-pi
  Sum : Sum  Inputs=|+-
  Sum1 : Sum  Inputs=|++
  SteerHWCmd : Outport
  wires:
  In1/1 -> Manual Switch/1, Sum/1
  Sum/1 -> Kp1/1, Ki/1, Kp/1  "error"
  Kp/1 -> Add/1
  In2/1 -> Sum/2
  Gain1/1 -> Manual Switch/2
  Add/1 -> Add1/1, Saturation/1
  Saturation/1 -> Add1/2, Gain1/1
  Ki/1 -> Sum1/1
  Sum1/1 -> Integrator/1
  Integrator/1 -> Add/3
  Ki1/1 -> Sum1/2
  Add1/1 -> Ki1/1
  Kp1/1 -> Derivative/1
  Derivative/1 -> Add/2
  Manual Switch/1 -> SteerHWCmd/1

== system MUDV_projekt/Environment/Ground Feedback ==
  Friction : Inport
  3D Engine : Subsystem  VariantControl=1
  Constant : Subsystem  VariantControl=0
  Ground : Outport  VectorParamsAs1DForOutWhenUnconnected=off

== system MUDV_projekt/Passenger Vehicle/Body, suspension and tires ==
  WindXYZ : Inport  Unit=m/s  PortDimensions=3
  Ground : Inport  Port=2  Unit=m  PortDimensions=4
  Friction : Inport  Port=3  Unit=1  PortDimensions=4
  WhlAng : Inport  Port=4  Unit=rad  PortDimensions=4
  AxlTrq : Inport  Port=5  Unit=N*m  PortDimensions=4
  BrkPrs : Inport  Port=6  PortDimensions=4
  Bus Selector : BusSelector  OutputSignals=InertFrm,BdyFrm  OutputAsBus=on
  Bus Selector1 : BusSelector  OutputSignals=TireFrame,Steering  OutputAsBus=on
  MacPherson Front Suspension Solid Axle Rear Suspension : Subsystem  VariantControl=3
      mask Display: image([imread('suspmacp.png');imread('suspsacoil.png')]);
  Vehicle : Subsystem
      mask Display: image('6dofcar.png');
  Wheels and Tires : Subsystem
      mask Display: image('wheel3dof.png')
  Bus Element Out3 : Outport  PortName=Veh
  Bus Element Out1 : Outport  Port=2  PortName=Wheels
  wires:
  Bus Selector/1 -> Bus Element Out3/1
  Wheels and Tires/2(Wheels2Susp) -> MacPherson Front Suspension Solid Axle Rear Suspension/3(Wheel)
  Bus Selector1/1 -> Bus Element Out1/1
  Ground/1 -> Wheels and Tires/5(Ground Input)
  BrkPrs/1 -> Wheels and Tires/4(Brake Press)
  Wheels and Tires/1(Wheels) -> Bus Selector1/1  "Wheels"
  Friction/1 -> Wheels and Tires/6(Friction)
  WindXYZ/1 -> Vehicle/2(Wind)
  Vehicle/1(VehFdbk) -> MacPherson Front Suspension Solid Axle Rear Suspension/2(Vehicle), Wheels and Tires/1(Veh), Bus Selector/1  "Veh"
  AxlTrq/1 -> Wheels and Tires/3(Axle Torque)
  WhlAng/1 -> MacPherson Front Suspension Solid Axle Rear Suspension/1(Steering)
  MacPherson Front Suspension Solid Axle Rear Suspension/1(Suspension) -> Wheels and Tires/2(Suspension), Vehicle/1(Suspension)  "Susp"

== system MUDV_projekt/Passenger Vehicle/Chassis Input ==
  Env : Inport
  Driveline : Inport  Port=2
  Bus Selector1 : BusSelector  OutputSignals=Gnd.z.G_FL_z,Gnd.z.G_FR_z,Gnd.z.G_RL_z,Gnd.z.G_RR_z
  Bus Selector2 : BusSelector  OutputSignals=Wind
  Bus Selector3 : BusSelector  OutputSignals=Gnd.mu.mu_FL,Gnd.mu.mu_FR,Gnd.mu.mu_RL,Gnd.mu.mu_RR
  Bus Selector4 : BusSelector  OutputSignals=WhlAng,AxlTrq,BrkPrs
  Vector Concatenate : Concatenate  NumInputs=4
  Vector Concatenate1 : Concatenate  NumInputs=4
  Wind : Outport  VectorParamsAs1DForOutWhenUnconnected=off
  Gnd : Outport  Port=2  VectorParamsAs1DForOutWhenUnconnected=off
  mu : Outport  Port=3  VectorParamsAs1DForOutWhenUnconnected=off
  WhlAng : Outport  Port=4  VectorParamsAs1DForOutWhenUnconnected=off
  AxlTrq : Outport  Port=5  VectorParamsAs1DForOutWhenUnconnected=off
  BrkPrs : Outport  Port=6  VectorParamsAs1DForOutWhenUnconnected=off
  wires:
  Env/1 -> Bus Selector3/1, Bus Selector1/1, Bus Selector2/1
  Bus Selector2/1 -> Wind/1  "<Wind>"
  Bus Selector3/1 -> Vector Concatenate/1  "<mu_FL>"
  Bus Selector3/2 -> Vector Concatenate/2  "<mu_FR>"
  Bus Selector3/3 -> Vector Concatenate/3  "<mu_RL>"
  Bus Selector3/4 -> Vector Concatenate/4  "<mu_RR>"
  Vector Concatenate/1 -> mu/1
  Bus Selector1/1 -> Vector Concatenate1/1  "<G_FL_z>"
  Bus Selector1/2 -> Vector Concatenate1/2  "<G_FR_z>"
  Bus Selector1/3 -> Vector Concatenate1/3  "<G_RL_z>"
  Bus Selector1/4 -> Vector Concatenate1/4  "<G_RR_z>"
  Vector Concatenate1/1 -> Gnd/1
  Driveline/1 -> Bus Selector4/1
  Bus Selector4/2 -> AxlTrq/1  "<AxlTrq>"
  Bus Selector4/1 -> WhlAng/1  "<WhlAng>"
  Bus Selector4/3 -> BrkPrs/1  "<BrkPrs>"

== system MUDV_projekt/Passenger Vehicle/Chassis Output ==
  Veh : Inport
  Wheels : Inport  Port=2
  Out Bus Element4 : Outport  PortName=VehFdbk
  Out Bus Element1 : Outport  Port=2  PortName=WheelsFdbk
  wires:
  Veh/1 -> Out Bus Element4/1
  Wheels/1 -> Out Bus Element1/1

== system MUDV_projekt/Passenger Vehicle/Driveline ==
  SteerHWCmd : Inport
  AxlTrqCmd : Inport  Port=2
  BrkPrsCmd : Inport  Port=3  PortDimensions=4
  Brake Hydraulics : Subsystem
  Ground3 : Ground
  Kinematic Steering : vehdynlibsteering/Kinematic Steering  StrgType=Ackerman  StrgRatioType=Constant  Loc=Front  NrmlFctr=1  TrckWdth=1.922  WhlBase=(1.515+1.504)  Db=0  StrgRng=3*pi  StrgAngBpts="[-6.2832   -5.0265   -3.7699   -2.5133   -1.2566         0    1.2566    2.5133    3.7699    5.0265    6.2832]"  StrgRatioTbl=|  StrgRatio=18  PctAckIn=off  PctAck=100  PctAckTbl=ones(1,11)*100  StrgArmLngth=0.1  RckCsLngth=0.5  TieRodLngth=0.248128028933392  D=0.2  PnnRadius=0.0057  PnnRadiusTbl="[0.0055    0.0055    0.0056    0.0057    0.0057    0.0057    0.0057    0.0057    0.0056    0.0055    0.0055]"  RodLngth=0.1  ParaArmLngth=0.9  aMode=2
      | [13.5000   13.3750   13.2500   13.1250   13.0000   13.0000   13.0000   13.1250   13.2500   13.3750   13.5000
      | ]
  Terminator : Terminator
  Torque Split : Subsystem
  Vector Concatenate : Concatenate
  Vector Concatenate1 : Concatenate
  Vector Concatenate2 : Concatenate
  WhlAng : Outport  Unit=rad  VectorParamsAs1DForOutWhenUnconnected=off
  AxlTrq : Outport  Port=2  VectorParamsAs1DForOutWhenUnconnected=off
  BrkPrs : Outport  Port=3  PortDimensions=4  VectorParamsAs1DForOutWhenUnconnected=off
  wires:
  Kinematic Steering/2 -> Vector Concatenate/1
  Vector Concatenate2/1 -> Vector Concatenate1/2  "RearWheelAngles"
  Vector Concatenate/1 -> Vector Concatenate1/1  "FrontWheelAngles"
  Ground3/1 -> Vector Concatenate2/2, Vector Concatenate2/1
  Vector Concatenate1/1 -> WhlAng/1
  Kinematic Steering/3 -> Vector Concatenate/2
  BrkPrsCmd/1 -> Brake Hydraulics/1(BrkPrsCmd)
  Kinematic Steering/1 -> Terminator/1
  Brake Hydraulics/1(BrkPrs) -> BrkPrs/1
  Torque Split/1(AxlTrq) -> AxlTrq/1
  AxlTrqCmd/1 -> Torque Split/1(AxlTrqCmd)
  SteerHWCmd/1 -> Kinematic Steering/1

== system MUDV_projekt/Passenger Vehicle/Driveline Input ==
  Controller : Inport
  Bus Selector1 : BusSelector  OutputSignals=signal2
  Bus Selector2 : BusSelector  OutputSignals=BrkPrsCmd
  Bus Selector3 : BusSelector  OutputSignals=signal1
  Steer : Outport  VectorParamsAs1DForOutWhenUnconnected=off
  AxlTrqCmd : Outport  Port=2  VectorParamsAs1DForOutWhenUnconnected=off
  BrkPrsCmd : Outport  Port=3  VectorParamsAs1DForOutWhenUnconnected=off
  wires:
  Bus Selector1/1 -> Steer/1  "<signal2>"
  Bus Selector3/1 -> AxlTrqCmd/1  "<signal1>"
  Bus Selector2/1 -> BrkPrsCmd/1  "<BrkPrsCmd>"
  Controller/1 -> Bus Selector2/1, Bus Selector3/1, Bus Selector1/1

== system MUDV_projekt/Passenger Vehicle/Driveline Output ==
  WhlAng : Inport
  AxlTrq : Inport  Port=2
  BrkPrs : Inport  Port=3
  Bus Creator1 : BusCreator  Inputs=3
  Driveline : Outport  VectorParamsAs1DForOutWhenUnconnected=off
  wires:
  Bus Creator1/1 -> Driveline/1  "Driveline"
  AxlTrq/1 -> Bus Creator1/2  "AxlTrq"
  WhlAng/1 -> Bus Creator1/1  "WhlAng"
  BrkPrs/1 -> Bus Creator1/3  "BrkPrs"

== system MUDV_projekt/Visualization/3D Engine ==
  note: 1) Add Subsystem or Model blocks as valid variant choices.
      | 2) You cannot connect blocks at this level. At simulation, connectivity is automatically
      | determined, based on the active variant and port name matching.
  VehFdbk : Inport
  3D Engine : Subsystem  VariantControl=engine3D==1
  3D Engine Disabled : Subsystem  VariantControl=engine3D==2

== system MUDV_projekt/Environment/Ground Feedback/3D Engine ==
  Friction : Inport
  Bus Creator : BusCreator  Inputs=4
  Bus Creator2 : BusCreator  Inputs=4
  Bus Creator3 : BusCreator  Inputs=2
  Bus Selector : BusSelector  OutputSignals=HitLoc
  Data Type Conversion : DataTypeConversion  SaturateOnIntegerOverflow=off  RndMeth=Floor
  Demux : Demux
  Demux1 : Demux
  First Order Hold : FirstOrderHold  ErrorTolerance=1
  Passenger Vehicle Ray Trace Set : sim3dlib/Vehicle Terrain Sensor  Priority=1  ActorTag=SimulinkVehicle1  VehExtEn=Constant  TireRadiiExt=Constant  VehCntrLngthVal=0  TireRadiiVal=0  VehRayLngth=10  LfRayLngth=20  RfRayLngth=20  LrRayLngth=20  RrRayLngth=20  VehRayOffset=0  LfRayOffset=-1  RfRayOffset=-1  LrRayOffset=-1  RrRayOffset=-1  VehEn=on  LfEn=on  RfEn=on  LrEn=on  RrEn=on  DbgEn=off  Ts=.03  aMode=2
  Range Limiter : Saturate  UpperLimit=1e3  LowerLimit=-1e3  ZeroCross=off
  Reshape10 : Reshape  OutputDimensionality=Row vector (2-D)
  Selector1 : Selector  InputPortWidth=5  IndexOptions=Index vector (dialog)  Indices=[2:5]  OutputSizes=1
  Signal Specification : SignalSpecification  Unit=m
  Signal Specification1 : SignalSpecification  Unit=1
  Terminator1 : Terminator
  Terminator2 : Terminator
  Zend Select : Selector  NumberOfDimensions=2  InputPortWidth=3  IndexOptions=Select all,Index vector (dialog)  Indices=[1 3],3  OutputSizes=1,1
  Ground : Outport  VectorParamsAs1DForOutWhenUnconnected=off
  wires:
  Zend Select/1 -> Reshape10/1
  Bus Selector/1 -> Range Limiter/1  "<HitLoc>"
  Passenger Vehicle Ray Trace Set/2 -> Terminator1/1
  Passenger Vehicle Ray Trace Set/3 -> Terminator2/1
  Reshape10/1 -> Selector1/1
  Passenger Vehicle Ray Trace Set/1 -> Bus Selector/1
  Selector1/1 -> Data Type Conversion/1
  Demux/2 -> Bus Creator/2  "G_FR_z"
  Demux/1 -> Bus Creator/1  "G_FL_z"
  Demux/4 -> Bus Creator/4  "G_RR_z"
  Demux/3 -> Bus Creator/3  "G_RL_z"
  Signal Specification/1 -> Demux/1
  Signal Specification1/1 -> Demux1/1
  Demux1/1 -> Bus Creator2/1  "mu_FL"
  Bus Creator/1 -> Bus Creator3/1  "z"
  Demux1/3 -> Bus Creator2/3  "mu_RL"
  Demux1/4 -> Bus Creator2/4  "mu_RR"
  Demux1/2 -> Bus Creator2/2  "mu_FR"
  Bus Creator2/1 -> Bus Creator3/2  "mu"
  Bus Creator3/1 -> Ground/1
  Range Limiter/1 -> Zend Select/1
  First Order Hold/1 -> Signal Specification/1
  Data Type Conversion/1 -> First Order Hold/1
  Friction/1 -> Signal Specification1/1

== system MUDV_projekt/Environment/Ground Feedback/Constant ==
  Friction : Inport
  Bus Creator : BusCreator  Inputs=4
  Bus Creator2 : BusCreator  Inputs=4
  Bus Creator3 : BusCreator  Inputs=2
  Constant1 : Constant  Value=zeros(4,1)
  Demux : Demux
  Demux1 : Demux
  Signal Specification : SignalSpecification  Unit=m
  Signal Specification1 : SignalSpecification  Unit=1
  Ground : Outport  VectorParamsAs1DForOutWhenUnconnected=off
  wires:
  Constant1/1 -> Signal Specification/1
  Signal Specification/1 -> Demux/1
  Demux/4 -> Bus Creator/4  "G_RR_z"
  Demux/1 -> Bus Creator/1  "G_FL_z"
  Demux/3 -> Bus Creator/3  "G_RL_z"
  Demux/2 -> Bus Creator/2  "G_FR_z"
  Bus Creator/1 -> Bus Creator3/1  "z"
  Demux1/3 -> Bus Creator2/3  "mu_RL"
  Demux1/4 -> Bus Creator2/4  "mu_RR"
  Demux1/1 -> Bus Creator2/1  "mu_FL"
  Demux1/2 -> Bus Creator2/2  "mu_FR"
  Bus Creator2/1 -> Bus Creator3/2  "mu"
  Friction/1 -> Signal Specification1/1
  Signal Specification1/1 -> Demux1/1
  Bus Creator3/1 -> Ground/1

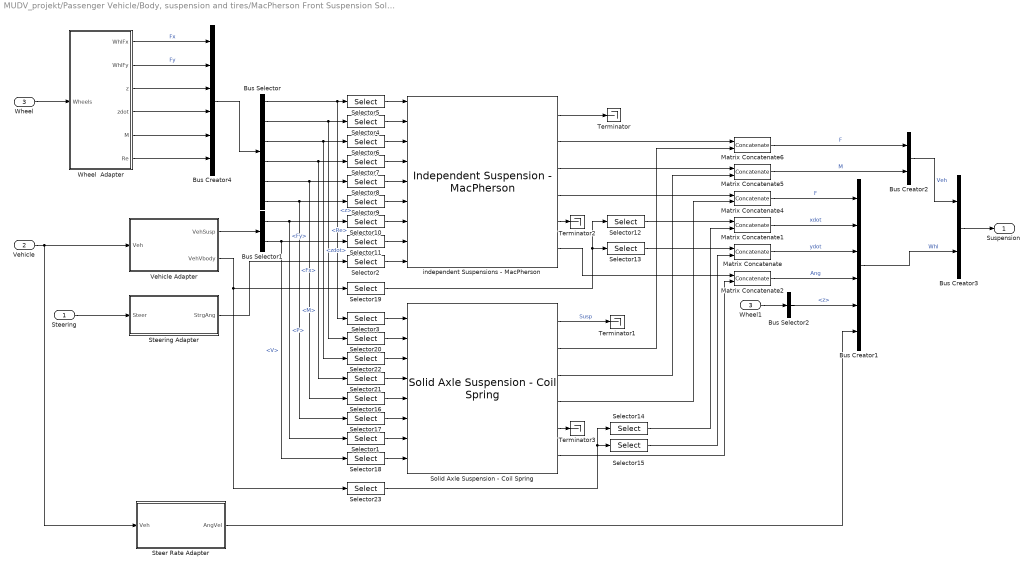
== system MUDV_projekt/Passenger Vehicle/Body, suspension and tires/MacPherson Front Suspension Solid Axle Rear Suspension ==
  Steering : Inport
  Vehicle : Inport  Port=2
  Wheel : Inport  Port=3
  Bus Creator1 : BusCreator  Inputs=6
  Bus Creator2 : BusCreator  Inputs=2
  Bus Creator3 : BusCreator  Inputs=2
  Bus Creator4 : BusCreator  Inputs=6
  Bus Selector : BusSelector  OutputSignals=z,Re,zdot,Fx,Fy,M
  Bus Selector1 : BusSelector  OutputSignals=P,V
  Bus Selector2 : BusSelector  OutputSignals=SuspFrame.z
  Matrix Concatenate{,1..2,4..6} (6 alike) : Concatenate  Mode=Multidimensional array  ConcatenateDimension=2
  Selector{1,17..18,23} (4 alike) : Selector  NumberOfDimensions=2  IndexOptions=Select all,Index vector (dialog)  Indices=[1 2],[3 4]  OutputSizes=1,1
  Selector{9..11,19} (4 alike) : Selector  NumberOfDimensions=2  IndexOptions=Select all,Index vector (dialog)  Indices=[1 2],[1 2]  OutputSizes=1,1
  Selector12 : Selector  NumberOfDimensions=2  InputPortWidth=3  IndexOptions=Index vector (dialog),Select all  Indices=1,1  OutputSizes=1,1
  Selector13 : Selector  NumberOfDimensions=2  InputPortWidth=3  IndexOptions=Index vector (dialog),Select all  Indices=2,1  OutputSizes=1,1
  Selector14 : Selector  NumberOfDimensions=2  InputPortWidth=3  IndexOptions=Index vector (dialog),Select all  Indices=1,1  OutputSizes=1,1
  Selector15 : Selector  NumberOfDimensions=2  InputPortWidth=3  IndexOptions=Index vector (dialog),Select all  Indices=2,1  OutputSizes=1,1
  Selector{3,16,20..22} (5 alike) : Selector  IndexOptions=Index vector (dialog)  Indices=[3 4]  OutputSizes=1
  Selector{2,4..8} (6 alike) : Selector  IndexOptions=Index vector (dialog)  Indices=[1 2]  OutputSizes=1
  Solid Axle Suspension - Coil Spring : vehdynlibsuspension/Solid Axle Suspension - Coil Spring  NumAxl=1  NumWhlsByAxl=2  StrgEnByAxl=0  WhlNumVec="[1  2]"  AxleNumVec="[1  1]"  SuspTypesByAxle=[1]  SuspImage=suspsacoil.png  AxlIxx=AxlIxx  AxlM=AxlM  TrackCoords=[0 0;VEH.TrackWidth*[-1 1]/2;0 0]  SuspCoords=[0 0;VEH.TrackWidth*[-1 1]/2;0 0]  KzWhlAxl=KzWhlAxl  F0zWhlAxl=F0zWhlAxl  CzWhlAxl=CzWhlAxl  IdealSuspEn=on  IdealSuspAxles=[1]  Kz=Kz  F0z=F0z(2)  Cz=Cz  Hmax=Hmax  Toe=0.  RollStrgSlp=0.  ToeStrgSlp=0  Caster=0.  CasterHslp=0.  CasterStrgSlp=0.01  Camber=0.  CamberHslp=0.  CamberStrgSlp=0.01  StrgHgtSlp=0.1432  MappedSuspEn=off  MappedSuspAxles="[1  2]"  f_susp_axl_bp=[1 2]  f_susp_dz_bp=[-0.15 -0.14 -0.13 -0.12 -0.11 -0.10 -0.09 -0.08 -0.07 -0.06 -0.05 -0.04 -0.03 -0.02 -0.01 0.00 0.01 0.02 0.03 0.04 0.05 0.06 0.07 0.08 0.09 0.10 0.11 0.12 0.13 0.14 0.15]  f_susp_dzdot_bp=[-0.15 -0.14 -0.13 -0.12 -0.11 -0.10 -0.09 -0.08 -0.07 -0.06 -0.05 -0.04 -0.03 -0.02 -0.01 0.00 0.01 0.02 0.03 0.04 0.05 0.06 0.07 0.08 0.09 0.10 0.11 0.12 0.13 0.14 0.15]  f_susp_fmz=zeros(31,31,61,2,4)  f_susp_geom=zeros(31,61,2,3)  f_susp_strgdelta_bp=[-30,-29,-28,-27,-26,-25,-24,-23,-22,-21,-20,-19,-18,-17,-16,-15,-14,-13,-12,-11,-10,-9,-8,-7,-6,-5,-4,-3,-2,-1,0,1,2,3,4,5,6,7,8,9,10,11,12,13,14,15,16,17,18,19,20,21,22,23,24,25,26,27,28,29,30]
  Steer Rate Adapter : Subsystem
  Steering Adapter : Subsystem
  Terminator{,1..3} (4 alike) : Terminator
  Vehicle Adapter : Subsystem
  Wheel  Adapter : Subsystem
  Wheel1 : InportShadow  Port=3
  independent Suspensions - MacPherson : vehdynlibsuspension/Independent Suspension - MacPherson  ActiveDampEn=off  NumAxl=1  NumWhlsByAxl=2  StrgEnByAxl=1  AntiSwayEnByAxl=1  WhlNumVec="[1  2]"  AxleNumVec="[1  1]"  SuspTypesByAxle=[1]  SuspImage=suspmacp.png  IdealSuspEn=on  IdealSuspAxles=[1]  Kz=Kz  F0z=F0z(1)  Cz=Cz  Hmax=Hmax  f_act_susp_cz=[10000 10000;10000 10000]  f_act_susp_duty_bpt=[0 1]  f_act_susp_zdot_bpt=[-1 1]  Toe=0.  RollStrgSlp=0.  ToeStrgSlp=0.  Caster=0.  CasterHslp=0.  CasterStrgSlp=0.  Camber=0.  CamberHslp=0.  CamberStrgSlp=0.  StrgHgtSlp=0.1432  MappedSuspEn=off  MappedSuspAxles="[1  2]"  f_susp_axl_bp=[1 2]  f_susp_dz_bp=[-0.15 -0.14 -0.13 -0.12 -0.11 -0.10 -0.09 -0.08 -0.07 -0.06 -0.05 -0.04 -0.03 -0.02 -0.01 0.00 0.01 0.02 0.03 0.04 0.05 0.06 0.07 0.08 0.09 0.10 0.11 0.12 0.13 0.14 0.15]  f_susp_dzdot_bp=[-0.15 -0.14 -0.13 -0.12 -0.11 -0.10 -0.09 -0.08 -0.07 -0.06 -0.05 -0.04 -0.03 -0.02 -0.01 0.00 0.01 0.02 0.03 0.04 0.05 0.06 0.07 0.08 0.09 0.10 0.11 0.12 0.13 0.14 0.15]  f_susp_fmz=zeros(31,31,61,2,4)  f_susp_geom=zeros(31,61,2,3)  f_susp_strgdelta_bp=[-30,-29,-28,-27,-26,-25,-24,-23,-22,-21,-20,-19,-18,-17,-16,-15,-14,-13,-12,-11,-10,-9,-8,-7,-6,-5,-4,-3,-2,-1,0,1,2,3,4,5,6,7,8,9,10,11,12,13,14,15,16,17,18,19,20,21,22,23,24,25,26,27,28,29,30]  AntiSwayR=0.2  AntiSwayNtrlAng=0.5236  AntiSwayTrsK=8e+02
  Suspension : Outport  VectorParamsAs1DForOutWhenUnconnected=off
  wires:
  Bus Creator3/1 -> Suspension/1
  Bus Creator1/1 -> Bus Creator3/2  "Whl"
  Bus Selector1/2 -> Selector11/1, Selector18/1  "<V>"
  Bus Selector/6 -> Selector9/1, Selector17/1  "<M>"
  Bus Selector/5 -> Selector8/1, Selector16/1  "<Fy>"
  Bus Selector/1 -> Selector3/1, Selector5/1  "<z>"
  Steering/1 -> Steering Adapter/1(Steer)
  Bus Selector1/1 -> Selector10/1, Selector1/1  "<P>"
  Matrix Concatenate/1 -> Bus Creator1/3  "ydot"
  independent Suspensions - MacPherson/6 -> Matrix Concatenate2/1
  Selector12/1 -> Matrix Concatenate1/1
  independent Suspensions - MacPherson/4 -> Matrix Concatenate4/1
  independent Suspensions - MacPherson/1 -> Terminator/1
  Bus Selector/4 -> Selector7/1, Selector21/1  "<Fx>"
  Vehicle Adapter/1(VehSusp) -> Bus Selector1/1
  independent Suspensions - MacPherson/2 -> Matrix Concatenate6/1
  independent Suspensions - MacPherson/3 -> Matrix Concatenate5/1
  Bus Creator2/1 -> Bus Creator3/1  "Veh"
  Steering Adapter/1(StrgAng) -> Selector2/1
  Bus Creator4/1 -> Bus Selector/1
  Wheel  Adapter/2(WhlFy) -> Bus Creator4/2  "Fy"
  Wheel  Adapter/1(WhlFx) -> Bus Creator4/1  "Fx"
  Wheel/1 -> Wheel  Adapter/1(Wheels)
  Wheel  Adapter/3(z) -> Bus Creator4/3
  Wheel  Adapter/4(zdot) -> Bus Creator4/4
  Wheel  Adapter/5(M) -> Bus Creator4/5
  Bus Selector/2 -> Selector20/1, Selector4/1  "<Re>"
  Selector2/1 -> independent Suspensions - MacPherson/9
  Selector3/1 -> Solid Axle Suspension - Coil Spring/1
  Selector4/1 -> independent Suspensions - MacPherson/2
  Selector5/1 -> independent Suspensions - MacPherson/1
  Selector6/1 -> independent Suspensions - MacPherson/3
  Selector7/1 -> independent Suspensions - MacPherson/4
  Selector8/1 -> independent Suspensions - MacPherson/5
  Selector9/1 -> independent Suspensions - MacPherson/6
  Selector10/1 -> independent Suspensions - MacPherson/7
  Selector11/1 -> independent Suspensions - MacPherson/8
  Selector13/1 -> Matrix Concatenate/1
  Selector15/1 -> Matrix Concatenate/2
  Matrix Concatenate1/1 -> Bus Creator1/2  "xdot"
  Selector14/1 -> Matrix Concatenate1/2
  Matrix Concatenate2/1 -> Bus Creator1/4  "Ang"
  Solid Axle Suspension - Coil Spring/6 -> Matrix Concatenate2/2
  Matrix Concatenate4/1 -> Bus Creator1/1  "F"
  Solid Axle Suspension - Coil Spring/4 -> Matrix Concatenate4/2
  Matrix Concatenate5/1 -> Bus Creator2/2  "M"
  Matrix Concatenate6/1 -> Bus Creator2/1  "F"
  Solid Axle Suspension - Coil Spring/2 -> Matrix Concatenate6/2
  Selector16/1 -> Solid Axle Suspension - Coil Spring/5
  Selector17/1 -> Solid Axle Suspension - Coil Spring/6
  Selector1/1 -> Solid Axle Suspension - Coil Spring/7
  Selector18/1 -> Solid Axle Suspension - Coil Spring/8
  Selector20/1 -> Solid Axle Suspension - Coil Spring/2
  Wheel  Adapter/6(Re) -> Bus Creator4/6
  Selector21/1 -> Solid Axle Suspension - Coil Spring/4
  Solid Axle Suspension - Coil Spring/3 -> Matrix Concatenate5/2
  Vehicle/1 -> Vehicle Adapter/1(Veh), Steer Rate Adapter/1(Veh)
  Selector22/1 -> Solid Axle Suspension - Coil Spring/3
  Bus Selector/3 -> Selector22/1, Selector6/1  "<zdot>"
  Solid Axle Suspension - Coil Spring/1 -> Terminator1/1  "Susp"
  Vehicle Adapter/2(VehVbody) -> Selector23/1, Selector19/1
  Steer Rate Adapter/1(AngVel) -> Bus Creator1/6
  independent Suspensions - MacPherson/5 -> Terminator2/1
  Solid Axle Suspension - Coil Spring/5 -> Terminator3/1
  Selector19/1 -> Selector12/1, Selector13/1
  Selector23/1 -> Selector15/1, Selector14/1
  Wheel1/1 -> Bus Selector2/1
  Bus Selector2/1 -> Bus Creator1/5  "<z>"
